simulink model "automata_learning"  (R2022a)
settings: Solver=FixedStepAuto  StartTime=0.0  StopTime=10.0  FixedStep=0.05  RelTol=1e-3
(part 1 of 10)
settings Model: Creator=diego  LastModifiedBy=diego

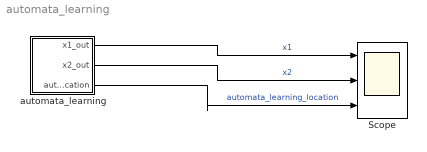
== system automata_learning ==
  Scope : Scope  NumInputPorts=3
  automata_learning : Stateflow chart  TreatAsAtomicUnit=on
  wires:
  automata_learning/1(x1_out) -> Scope/1  "x1"
  automata_learning/2(x2_out) -> Scope/2  "x2"
  automata_learning/3(automata_learning_location) -> Scope/3  "automata_learning_location"
